simulink model "Model1"  (R2023b)
settings: Solver=VariableStepAuto  StartTime=0.0  StopTime=10.0  RelTol=1e-3
settings Model: Creator=csj7701  LastModifiedBy=csj7701
settings DataIOCC: SaveFormat=Array

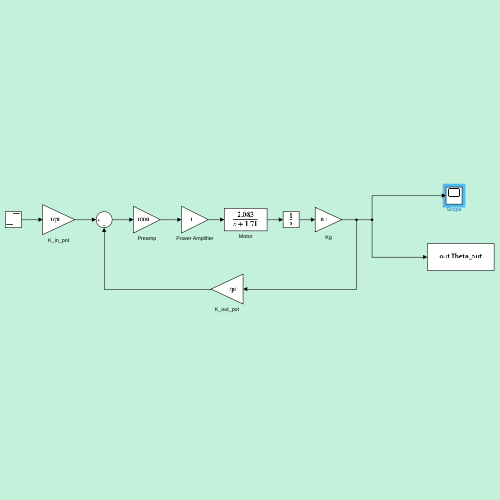
[thumbnail: Simulink's stored preview of the top-level diagram]
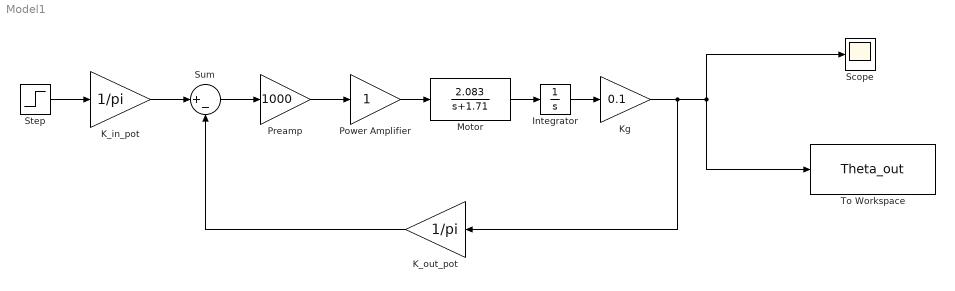
== system Model1 ==
  Integrator : Integrator
  K_in_pot : Gain  Gain=1/pi
  K_out_pot : Gain  Gain=1/pi
  Kg : Gain  Gain=0.1
  Motor : TransferFcn  Numerator=[2.083]  Denominator=[1 1.71]
  Power Amplifier : Gain
  Preamp : Gain  Gain=1000
  Scope : Scope
  Step : Step  Time=0  After=30  SampleTime=0
  Sum : Sum  Inputs=|+-
  To Workspace : ToWorkspace  VariableName=Theta_out  SampleTime=-1
  wires:
  K_in_pot/1 -> Sum/1
  Step/1 -> K_in_pot/1
  Sum/1 -> Preamp/1
  Preamp/1 -> Power Amplifier/1
  Power Amplifier/1 -> Motor/1
  Motor/1 -> Integrator/1
  Integrator/1 -> Kg/1
  Kg/1 -> K_out_pot/1, Scope/1, To Workspace/1
  K_out_pot/1 -> Sum/2
